simulink model "exercise_fixedpoint_2008b"  (Simulink 7.2)
settings: Solver=VariableStepDiscrete  StartTime=0.0  StopTime=1  RelTol=1e-3
libraries: simulink x1
settings Model: Creator=morgy  LastModifiedBy=morgy
settings DebuggingCC: FcnCallInpInsideContextMsg=Enable All  StrictBusMsg=ErrorLevel1
settings GRTTargetCC: CombineOutputUpdateFcns=on

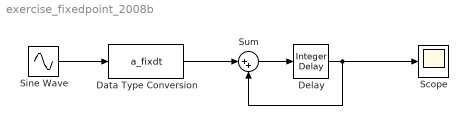
== system exercise_fixedpoint_2008b ==
  Data Type Conversion : DataTypeConversion  OutDataTypeStr=a_fixdt  OutDataTypeMode=Specify via dialog  OutDataType=a_fixdt  LockScale=on
  Delay : simulink/Discrete/Integer Delay  NumDelays=1  vinit=0  samptime=-1
  Scope : Scope
  Sine Wave : Sin  Frequency=2*pi*100  SampleTime=1/48000
  Sum : Sum  Inputs=|++  AccumDataTypeStr=a_fixdt
  wires:
  Sum/1 -> Delay/1
  Sine Wave/1 -> Data Type Conversion/1
  Delay/1 -> Scope/1, Sum/2
  Data Type Conversion/1 -> Sum/1
